simulink model "barriereTrainv2"  (R2021a)
settings: Solver=ode15s  StartTime=0.0  StopTime=100.0  FixedStep=0.1  RelTol=1e-3  EnableMultiTasking=on
settings Model: Creator=M1  LastModifiedBy=alvic
settings SolverCC: AlgebraicLoopSolver=TrustRegion  AutoInsertRateTranBlk=on
settings DataIOCC: LimitDataPoints=on  ReturnWorkspaceOutputs=off
settings OptimizationCC: LifeSpan=inf
settings DebuggingCC: AllowSymbolicDim=off  SFUnexpectedBacktrackingDiag=warning  SFNoUnconditionalDefaultTransitionDiag=warning  SFExecutionAtInitializationDiag=none  SFMachineParentedDataDiag=warning  ArithmeticOperatorsInVariantConditions=warning
settings SFSimCC: SimUseLocalCustomCode=off  CustomCodeUndefinedFunction=UseInterfaceOnly
settings RTWCC: RTWUseLocalCustomCode=off
settings CodeAppCC: StateflowObjectComments=on
settings GRTTargetCC: TargetLangStandard=C89/C90 (ANSI)
settings ConfigComp: CovMetricSettings=dw  CovSaveCumulativeToWorkspaceVar=on  CovSaveSingleToWorkspaceVar=on  CovExternalEMLEnable=off  CovSFcnEnable=off

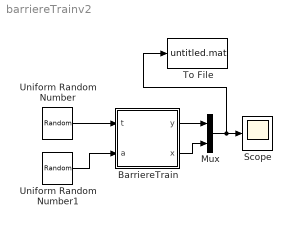
== system barriereTrainv2 ==
  BarriereTrain : Stateflow chart  TreatAsAtomicUnit=on
  Mux : Mux  Inputs=2
  Scope : Scope
  To File : ToFile  SaveFormat=Timeseries
  Uniform Random Number : UniformRandomNumber  Minimum=3  Maximum=15  Seed=2  SampleTime=1
  Uniform Random Number1 : UniformRandomNumber  Minimum=-500  Maximum=-400  SampleTime=1
  wires:
  Uniform Random Number1/1 -> BarriereTrain/2(a)
  Uniform Random Number/1 -> BarriereTrain/1(t)
  BarriereTrain/1(y) -> Mux/1
  BarriereTrain/2(x) -> Mux/2
  Mux/1 -> To File/1, Scope/1

== stateflow chart barriereTrainv2/BarriereTrain ==
  settings: updateMethod=CONTINUOUS
  state train [parallel]
    settings: executionOrder=1
    state Far
      during :
      x_dot = decc;
      1000 <= x;
    state Near
      during :
      x_dot = decc+300;
      0 <= x;
    state No_train
      x_dot = 0;
    state Past
      during :
      x_dot = a;
      -150 <= x;
    note: On considère que x est la position du train et
        | y la position de la barrière
    (default) -> Far : {decc = a}
    Far -> Near : [x<1000]
    Near -> Past : [x < 0]
    No_train -> Far : [after(t, sec)]{x = 5000}
    Past -> No_train : [x <= -150]{decc = a}
  state barriere [parallel]
    settings: executionOrder=3
    note: La barrière est ouverte pour y = 90
    state moveup
      during :
      y_dot = 40;
    state open
      during :
      y_dot = 0;
    state movedown
      during :
      y_dot = -40;
    state closed
    note: La porte est fermée pour y = 0
    (default) -> open
    moveup -> open [order 1] : [y >= 90]
    closed -> moveup : [in(controleur.Mont)]
    open -> movedown : [in(controleur.Desc)]
    movedown -> moveup [order 2] : [in(controleur.Mont)]
    moveup -> movedown [order 2] : [in(controleur.Desc)]
    movedown -> closed [order 1] : [y <= 0]
  state controleur [parallel]
    settings: executionOrder=2
    note: Le contrôleur supervise la commande de la
        | barrière en fonction de la position du train
    state Tempo
    state Mont
    state idle
    state Desc
    Tempo -> Mont : [after(2, sec)]
    Desc -> Tempo : [in(train.No_train) || in(train.Past)]
    (default) -> idle
    Mont -> idle [order 1] : [in(train.Far)]
    Mont -> Desc [order 2] : [in(train.Near)]
    idle -> Desc : [in(train.Near)]
  data: t input double; y output =90; a input; x output =5000; decc local single
  data y settings: updateMethod=SF_CONTINUOUS_TIME_DATA
  data x settings: updateMethod=SF_CONTINUOUS_TIME_DATA
  data decc settings: updateMethod=SF_CONTINUOUS_TIME_DATA
